simulink model "sim2"  (R2024a)
settings: Solver=FixedStepAuto  StartTime=0.0  StopTime=20.0  FixedStep=1e-3  RelTol=1e-3
values from neighbouring files (symbols this model uses):
  zad1 =     [ident_lab2_v08.mat]
libraries: matrix_library x1
settings Model: Creator=alexe  LastModifiedBy=alexe

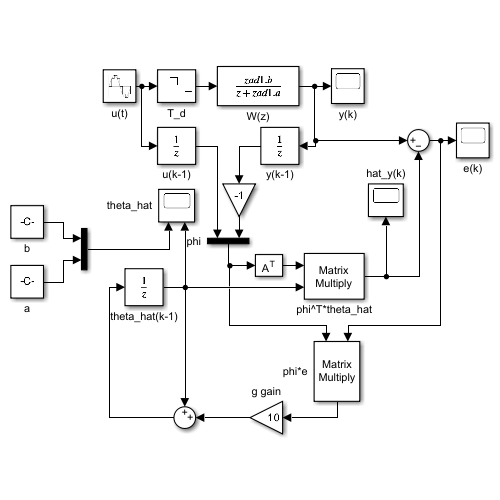
[thumbnail: Simulink's stored preview of the top-level diagram]
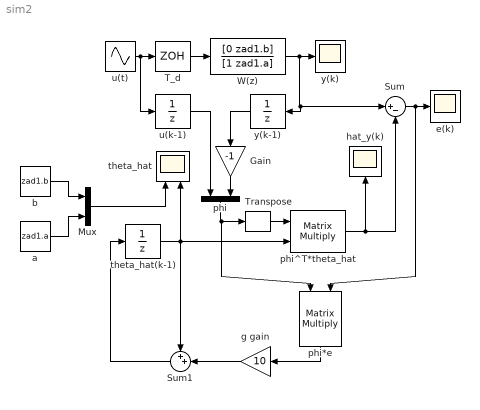
== system sim2 ==
  Gain : Gain  Gain=-1
  Mux : Mux  Inputs=2
  Sum : Sum  Inputs=|+-
  Sum1 : Sum  Inputs=++|
  T_d : ZeroOrderHold  SampleTime=0.1
  Transpose : matrix_library/Transpose
  W(z) : DiscreteTransferFcn  Numerator=[0 zad1.b]  Denominator=[1 zad1.a]
  a : Constant  Value=zad1.a
  b : Constant  Value=zad1.b
  e(k) : Scope
  g gain : Gain  Gain=10
  hat_y(k) : Scope
  phi : Mux  Inputs=2
  phi*e : Product  Multiplication=Matrix(*)
  phi^T*theta_hat : Product  Multiplication=Matrix(*)
  theta_hat : Scope  NumInputPorts=2
  theta_hat(k-1) : UnitDelay  InitialCondition=[0;0];  SampleTime=0.1  HasFrameUpgradeWarning=on
  u(k-1) : UnitDelay  SampleTime=0.1  HasFrameUpgradeWarning=on
  u(t) : Sin  Frequency=zad1.w
  y(k) : Scope
  y(k-1) : UnitDelay  SampleTime=0.1  HasFrameUpgradeWarning=on
  wires:
  u(t)/1 -> u(k-1)/1, T_d/1
  T_d/1 -> W(z)/1
  W(z)/1 -> Sum/1, y(k-1)/1, y(k)/1
  u(k-1)/1 -> phi/1
  Gain/1 -> phi/2
  y(k-1)/1 -> Gain/1
  phi/1 -> Transpose/1, phi*e/1
  Transpose/1 -> phi^T*theta_hat/1
  theta_hat(k-1)/1 -> phi^T*theta_hat/2, Sum1/1, theta_hat/2
  phi^T*theta_hat/1 -> Sum/2, hat_y(k)/1
  Sum/1 -> phi*e/2, e(k)/1
  phi*e/1 -> g gain/1
  g gain/1 -> Sum1/2
  Sum1/1 -> theta_hat(k-1)/1
  b/1 -> Mux/1
  a/1 -> Mux/2
  Mux/1 -> theta_hat/1
